simulink model "test_integration"  (R2022b)
settings: Solver=FixedStepAuto  StartTime=0.0  StopTime=240  FixedStep=0.1  RelTol=1e-3
(part 1 of 2)
settings Model: Creator=rosit  LastModifiedBy=cristian
settings ConfigComp: CovScope=ReferencedModels  CovIncludeTopModel=off  CovHTMLOptions=-sRT=1 -sVT=0 -aTS=1 -agT=1 -bRG=1 -bTC=1 -hTR=0 -nFC=0 -nFD=1 -scm=1 -bcm=1 -xEv=0 -xEM=0 -req=1  CovEnableCumulative=off

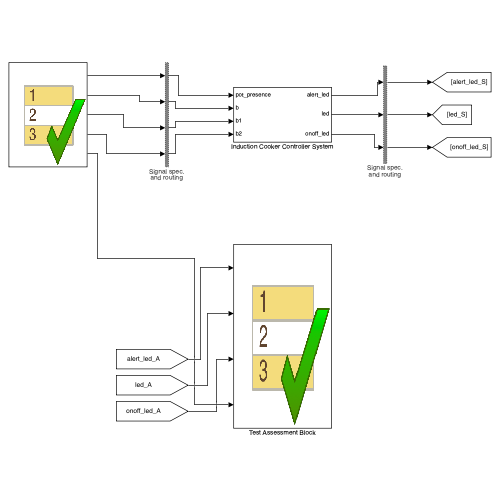
[thumbnail: Simulink's stored preview of the top-level diagram]
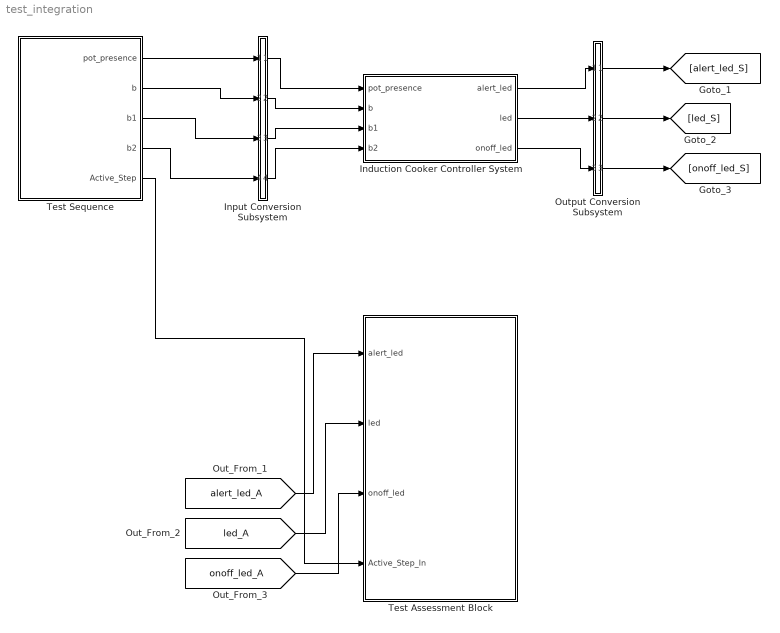
== system test_integration ==
  Induction Cooker Controller System : Subsystem
  Input Conversion Subsystem : Subsystem  Tag=__SLT_ICS__  Description=|
      | Signal spec.
      | and routing
      settings: AttributesFormatString=%<Description>
  Output Conversion Subsystem : Subsystem  Tag=__SLT_OCS__  Description=|
      | Signal spec.
      | and routing
      settings: AttributesFormatString=%<Description>
  Test Assessment Block : Test Sequence  Tag=__SLT_ASMT__  TreatAsAtomicUnit=on
  Test Sequence : Test Sequence  TreatAsAtomicUnit=on
  wires:
  [alert_led_A] -> Test Assessment Block/1(alert_led)
  [led_A] -> Test Assessment Block/2(led)
  [onoff_led_A] -> Test Assessment Block/3(onoff_led)
  Test Sequence/1(pot_presence) -> Input Conversion Subsystem/1(Inport_1)
  Test Sequence/2(b) -> Input Conversion Subsystem/2(Inport_2)
  Test Sequence/3(b1) -> Input Conversion Subsystem/3(Inport_3)
  Test Sequence/4(b2) -> Input Conversion Subsystem/4(Inport_4)
  Output Conversion Subsystem/1(Outport_1) -> [alert_led_S]
  Output Conversion Subsystem/2(Outport_2) -> [led_S]
  Output Conversion Subsystem/3(Outport_3) -> [onoff_led_S]
  Input Conversion Subsystem/1(Outport_1) -> Induction Cooker Controller System/1(pot_presence)
  Input Conversion Subsystem/2(Outport_2) -> Induction Cooker Controller System/2(b)
  Input Conversion Subsystem/3(Outport_3) -> Induction Cooker Controller System/3(b1)
  Input Conversion Subsystem/4(Outport_4) -> Induction Cooker Controller System/4(b2)
  Induction Cooker Controller System/1(alert_led) -> Output Conversion Subsystem/1(Inport_1)
  Induction Cooker Controller System/2(led) -> Output Conversion Subsystem/2(Inport_2)
  Induction Cooker Controller System/3(onoff_led) -> Output Conversion Subsystem/3(Inport_3)
  Test Sequence/5(Active_Step) -> Test Assessment Block/4(Active_Step_In)

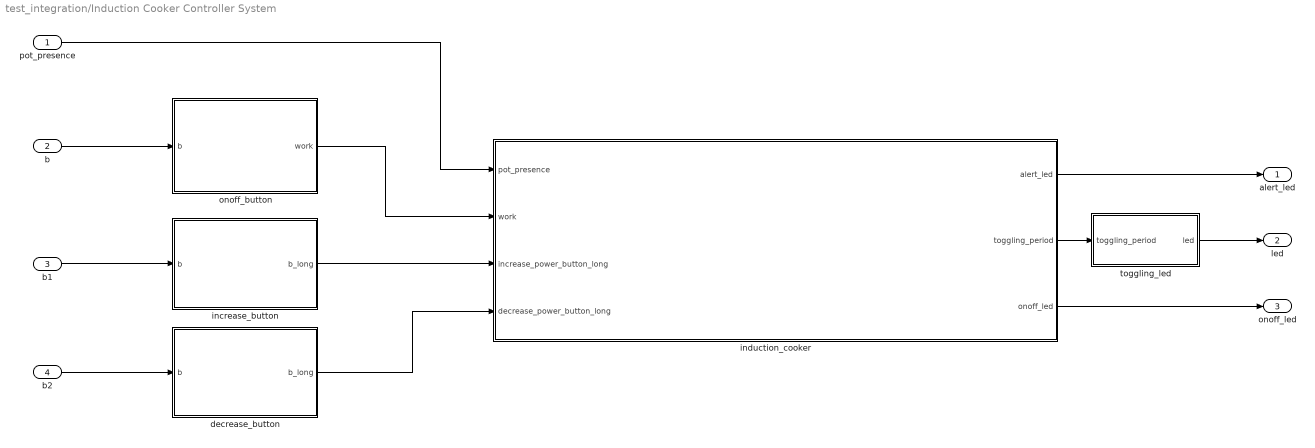
== system test_integration/Induction Cooker Controller System ==
  pot_presence : Inport
  b : Inport  Port=2
  b1 : Inport  Port=3
  b2 : Inport  Port=4
  decrease_button : Stateflow chart  TreatAsAtomicUnit=on
  increase_button : Stateflow chart  TreatAsAtomicUnit=on
  induction_cooker : Stateflow chart  TreatAsAtomicUnit=on
  onoff_button : Stateflow chart  TreatAsAtomicUnit=on
  toggling_led : Stateflow chart  TreatAsAtomicUnit=on
  alert_led : Outport
  led : Outport  Port=2
  onoff_led : Outport  Port=3
  wires:
  decrease_button/1(b_long) -> induction_cooker/4(decrease_power_button_long)
  increase_button/1(b_long) -> induction_cooker/3(increase_power_button_long)
  induction_cooker/2(toggling_period) -> toggling_led/1(toggling_period)
  toggling_led/1(led) -> led/1
  b1/1 -> increase_button/1(b)
  induction_cooker/3(onoff_led) -> onoff_led/1
  onoff_button/1(work) -> induction_cooker/2(work)
  b2/1 -> decrease_button/1(b)
  induction_cooker/1(alert_led) -> alert_led/1
  pot_presence/1 -> induction_cooker/1(pot_presence)
  b/1 -> onoff_button/1(b)

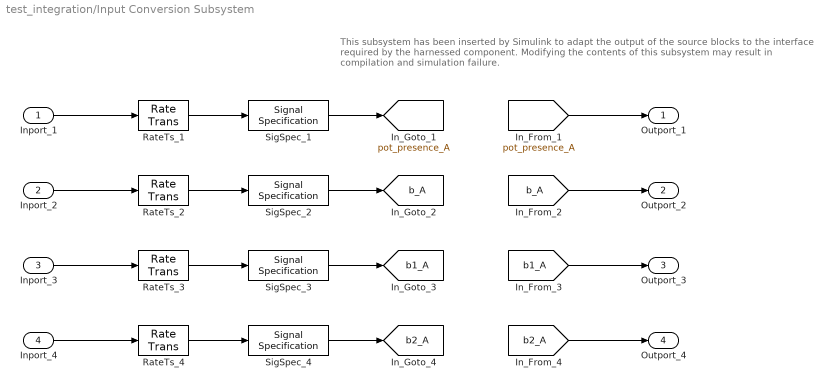
== system test_integration/Input Conversion Subsystem ==
  note: This subsystem has been inserted by Simulink to adapt the output of the source blocks to the interface required by the harnessed component.
      |  Modifying the contents of this subsystem may result in compilation and simulation failure.
  Inport_1 : Inport
  Inport_2 : Inport  Port=2
  Inport_3 : Inport  Port=3
  Inport_4 : Inport  Port=4
  RateTs_{1..4} (4 alike) : RateTransition  OutPortSampleTime=[-1, 0]
  SigSpec_{1..4} (4 alike) : SignalSpecification  OutDataTypeStr=boolean  Dimensions=[1]  SampleTime=[-1, 0]
  Outport_1 : Outport
  Outport_2 : Outport  Port=2
  Outport_3 : Outport  Port=3
  Outport_4 : Outport  Port=4
  tag scope: b1_A=global, b2_A=global, b_A=global, pot_presence_A=global
  wires:
  [pot_presence_A] -> Outport_1/1
  SigSpec_1/1 -> [pot_presence_A]
  RateTs_1/1 -> SigSpec_1/1
  Inport_1/1 -> RateTs_1/1
  [b_A] -> Outport_2/1
  SigSpec_2/1 -> [b_A]
  RateTs_2/1 -> SigSpec_2/1
  Inport_2/1 -> RateTs_2/1
  [b1_A] -> Outport_3/1
  SigSpec_3/1 -> [b1_A]
  RateTs_3/1 -> SigSpec_3/1
  Inport_3/1 -> RateTs_3/1
  [b2_A] -> Outport_4/1
  SigSpec_4/1 -> [b2_A]
  RateTs_4/1 -> SigSpec_4/1
  Inport_4/1 -> RateTs_4/1

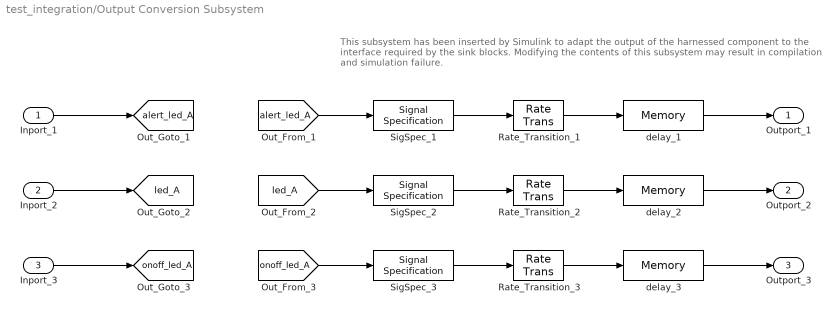
== system test_integration/Output Conversion Subsystem ==
  note: This subsystem has been inserted by Simulink to adapt the output of the harnessed component to the interface required by the sink blocks.
      |  Modifying the contents of this subsystem may result in compilation and simulation failure.
  Inport_1 : Inport
  Inport_2 : Inport  Port=2
  Inport_3 : Inport  Port=3
  Rate_Transition_1 : RateTransition  OutPortSampleTimeOpt=Inherit
  Rate_Transition_2 : RateTransition  OutPortSampleTimeOpt=Inherit
  Rate_Transition_3 : RateTransition  OutPortSampleTimeOpt=Inherit
  SigSpec_1 : SignalSpecification  OutDataTypeStr=boolean  Dimensions=[1]
  SigSpec_2 : SignalSpecification  OutDataTypeStr=boolean  Dimensions=[1]
  SigSpec_3 : SignalSpecification  OutDataTypeStr=boolean  Dimensions=[1]
  delay_1 : Memory
  delay_2 : Memory
  delay_3 : Memory
  Outport_1 : Outport
  Outport_2 : Outport  Port=2
  Outport_3 : Outport  Port=3
  tag scope: alert_led_A=global, led_A=global, onoff_led_A=global
  wires:
  Inport_1/1 -> [alert_led_A]
  [alert_led_A] -> SigSpec_1/1
  SigSpec_1/1 -> Rate_Transition_1/1
  Rate_Transition_1/1 -> delay_1/1
  delay_1/1 -> Outport_1/1
  Inport_2/1 -> [led_A]
  [led_A] -> SigSpec_2/1
  SigSpec_2/1 -> Rate_Transition_2/1
  Rate_Transition_2/1 -> delay_2/1
  delay_2/1 -> Outport_2/1
  Inport_3/1 -> [onoff_led_A]
  [onoff_led_A] -> SigSpec_3/1
  SigSpec_3/1 -> Rate_Transition_3/1
  Rate_Transition_3/1 -> delay_3/1
  delay_3/1 -> Outport_3/1

== stateflow chart test_integration/Induction Cooker Controller System/decrease_button ==
  note: Bottone a livelli, la pressione per un numero di secondi pari a DURATION permette di avere un uscita alta in maniera istantanea.
      | Per avere in output un valore PRESSED, è necessare lasciare il bottone e premere tra un output e l'altro.
  state Wait
    en: b_long = RELEASED
  state Pressed
    en: b_long = RELEASED;
    on after(DURATION,sec): b_long = PRESSED
  state LongPressed
    en: b_long = RELEASED
  (default) -> Wait
  Wait -> Pressed : [b == PRESSED]
  Pressed -> Wait [order 1] : [b == RELEASED]
  LongPressed -> Wait : [b == RELEASED]
  Pressed -> LongPressed [order 2] : [b_long == PRESSED && b == PRESSED]
  data: b_long output boolean size=1; PRESSED constant boolean size=1 =0; RELEASED constant boolean size=1 =1; b input boolean size=1; DURATION constant double size=1 =1

== stateflow chart test_integration/Induction Cooker Controller System/increase_button ==
  note: Bottone a livelli, la pressione per un numero di secondi pari a DURATION permette di avere un uscita alta in maniera istantanea.
      | Per avere in output un valore PRESSED, è necessare lasciare il bottone e premere tra un output e l'altro.
  state Wait
    en: b_long = RELEASED
  state Pressed
    en: b_long = RELEASED;
    on after(DURATION,sec): b_long = PRESSED
  state LongPressed
    en: b_long = RELEASED
  (default) -> Wait
  Wait -> Pressed : [b == PRESSED]
  Pressed -> Wait [order 1] : [b == RELEASED]
  LongPressed -> Wait : [b == RELEASED]
  Pressed -> LongPressed [order 2] : [b_long == PRESSED && b == PRESSED]
  data: b_long output boolean size=1; PRESSED constant boolean size=1 =0; RELEASED constant boolean size=1 =1; b input boolean size=1; DURATION constant double size=1 =1

== stateflow chart test_integration/Test Sequence ==
  settings: updateMethod=DISCRETE  sampleTime=0.1
  state IncreasePower
    state IP_Init
      %% Initialize data outputs.
      pot_presence = true;
      b = true;
      b1 = true;
      b2 = true;
      settings: description=Inizialmente il fornello è spento.
    state IP_TurnON
      pot_presence = true;
      b = false;
      b1 = true;
      b2 = true;
      settings: description=Accendiamo il fornello, premendo l'apposito pulsante di accensione. Il passaggio avveiene in maniera istantanea.
    state IP_IncreasePower300W
      pot_presence = false;
      b = true;
      b1 = false;
      b2 = true;
      settings: description=Posizioniamo la pentola ed accendiamo il fornello facendo pressione per 1 secondo sull'apposito pulsante di aumento potenza.
    state IP_Wait300W
      pot_presence = false;
      b = true;
      b1 = true;
      b2 = true;
      settings: description=Attendiamo 5 sec affinché il cambiamento diventi effettivo.
    state IP_Set300W
      pot_presence = false;
      b = true;
      b1 = true;
      b2 = true;
      settings: description=Il cambiamento di potenza viene effettuato.
    state IP_IncreasePower500W
      pot_presence = false;
      b = true;
      b1 = false;
      b2 = true;
      settings: description=Posizioniamo la pentola ed accendiamo il fornello facendo pressione per 1 secondo sull'apposito pulsante di aumento potenza.
    state IP_Wait500W
      pot_presence = false;
      b = true;
      b1 = true;
      b2 = true;
      settings: description=Attendiamo 5 sec affinché il cambiamento diventi effettivo.
    state IP_Set500W
      pot_presence = false;
      b = true;
      b1 = true;
      b2 = true;
      settings: description=Il cambiamento di potenza viene effettuato.
    state Void
    (default) -> IP_Init
    IP_Init -> IP_TurnON : [
        | true
        | ]
    IP_TurnON -> IP_IncreasePower300W : [
        | true
        | ]
    IP_IncreasePower300W -> IP_Wait300W : [
        | after(1+SamplePeriod,sec)
        | ]
    IP_Wait300W -> IP_Set300W : [
        | after(5-SamplePeriod,sec)
        | ]
    IP_Set300W -> IP_IncreasePower500W : [
        | true
        | ]
    IP_IncreasePower500W -> IP_Wait500W : [
        | after(1+SamplePeriod,sec)
        | ]
    IP_Wait500W -> IP_Set500W : [
        | after(5-SamplePeriod,sec)
        | ]
    IP_Set500W -> Void : [
        | true
        | ]
  state DecreasePower
    state DP_Init
      %% Initialize data outputs.
      pot_presence = true;
      b = true;
      b1 = true;
      b2 = true;
      settings: description=Inizialmente il fornello è spento.
    state DP_TurnON
      pot_presence = true;
      b = false;
      b1 = true;
      b2 = true;
      settings: description=Accendiamo il fornello, premendo l'apposito pulsante di accensione. Il passaggio avveiene in maniera istantanea.
    state DP_IncreasePower300W
      pot_presence = false;
      b = true;
      b1 = false;
      b2 = true;
      settings: description=Posizioniamo la pentola ed accendiamo il fornello facendo pressione per 1 secondo sull'apposito pulsante di aumento potenza.
    state DP_Wait300W
      pot_presence = false;
      b = true;
      b1 = true;
      b2 = true;
      settings: description=Attendiamo 5 sec affinché il cambiamento diventi effettivo.
    state DP_Set300W
      pot_presence = false;
      b = true;
      b1 = true;
      b2 = true;
      settings: description=Il cambiamento di potenza viene effettuato.
    state DP_DecreasePower0W
      pot_presence = false;
      b = true;
      b1 = true;
      b2 = false;
      settings: description=Facciamo pressione per 1 secondo sull'apposito pulsante di diminuzione di potenza.
    state DP_Wait0W
      pot_presence = false;
      b = true;
      b1 = true;
      b2 = true;
      settings: description=Attendiamo 5 sec affinché il cambiamento diventi effettivo.
    state DP_Set0W
      pot_presence = false;
      b = true;
      b1 = true;
      b2 = true;
      settings: description=Il cambiamento di potenza viene effettuato.
    state DP_void
    (default) -> DP_Init
    DP_Init -> DP_TurnON : [
        | true
        | ]
    DP_TurnON -> DP_IncreasePower300W : [
        | true
        | ]
    DP_IncreasePower300W -> DP_Wait300W : [
        | after(1+SamplePeriod,sec)
        | ]
    DP_Wait300W -> DP_Set300W : [
        | after(5-SamplePeriod,sec)
        | ]
    DP_Set300W -> DP_DecreasePower0W : [
        | true
        | ]
    DP_DecreasePower0W -> DP_Wait0W : [
        | after(1+SamplePeriod,sec)
        | ]
    DP_Wait0W -> DP_Set0W : [
        | after(5-SamplePeriod,sec)
        | ]
    DP_Set0W -> DP_void : [
        | true
        | ]
  state TurnOnOff
    state TO_Init
      %% Initialize data outputs.
      pot_presence = true;
      b = true;
      b1 = true;
      b2 = true;
      settings: description=All'inizio il fornello è spento e quindi anche il led di accensione.
    state TO_PowerOn
      pot_presence = true;
      b = false;
      b1 = true;
      b2 = true;
      settings: description=Dopodiché il bottone viene premuto ed il fornello si accende istantaneamente.
    state TO_Release
      pot_presence = true;
      b = true;
      b1 = true;
      b2 = true;
      settings: description=Quando il bottone viene rilasciato, il bottone ed il led di accensione sono entrambi accesi.
    state TO_PowerOff
      pot_presence = true;
      b = false;
      b1 = true;
      b2 = true;
      settings: description=Dopodiché il bottone viene ripremuto per la durata di un secondo ed il fornello, con il rispettivo led, vengono spenti.
    state TO_End
      pot_presence = true;
      b = true;
      b1 = true;
      b2 = true;
      settings: description=Infine il fornello è spento.
    state TO_Void
    (default) -> TO_Init
    TO_Init -> TO_PowerOn : [
        | true
        | ]
    TO_PowerOn -> TO_Release : [
        | true
        | ]
    TO_Release -> TO_PowerOff : [
        | true
        | ]
    TO_PowerOff -> TO_End : [
        | after(1+SamplePeriod,sec)
        | ]
    TO_End -> TO_Void : [
        | true
        | ]
  state PotRemovedWhileCooking
    state PR_Init
      %% Initialize data outputs.
      pot_presence = true;
      b = true;
      b1 = true;
      b2 = true;
      settings: description=inizialmente il fornello è spento.
    state PR_TurnOn
      pot_presence = true;
      b = false;
      b1 = true;
      b2 = true;
      settings: description=Accendiamo il fornello.
    state PR_IncreasePower300W
      pot_presence = false;
      b = true;
      b1 = false;
      b2 = true;
      settings: description=Pressione del bottone per incrementare la potenza da 0W a 300W.
    state PR_Wait300W
      pot_presence = false;
      b = true;
      b1 = true;
      b2 = true;
      settings: description=Attesa che il cambiamento di potenza sia effettivo per 5 sec.
    state PR_Set300W
      pot_presence = false;
      b = true;
      b1 = true;
      b2 = true;
      settings: description=Facciamo funzionare un po' il fornello.
    state PR_PotRemoved
      pot_presence = true;
      b = true;
      b1 = true;
      b2 = true;
      settings: description=|
          | La pentola viene rimossa dal fornello.
          | Si accende il led rosso.
    state PR_Alarm1
      pot_presence = true;
      b = true;
      b1 = true;
      b2 = true;
      settings: description=Il fornello è in stato di allarme, il led rosso è acceso
    state PR_PotPositioned
      pot_presence = false;
      b = true;
      b1 = true;
      b2 = true;
      settings: description=La pentola viene riposizionata, il led rosso si spegne, mentre il fornello continua a funzionare.
    state PR_ContinueWorking
      pot_presence = false;
      b = true;
      b1 = true;
      b2 = true;
      settings: description=Il fornello continua a funzionare normalmente per due secondi.
    state PR_PotRemoved2
      pot_presence = true;
      b = true;
      b1 = true;
      b2 = true;
      settings: description=La pentola viene rimossa e il fornello va immediatamente in tasto di allarme. Il led rosso si accende.
    state PR_Alarm2
      pot_presence = true;
      b = true;
      b1 = true;
      b2 = true;
      settings: description=Il fornello è instato di allarme, il led rosso è acceso.
    state PR_TimeElapsed
      pot_presence = true;
      b = true;
      b1 = true;
      b2 = true;
      settings: description=Il tempo di allarme è scaduto, il led rosso si è spento, il fornello è acceso, ma non sta funzionando (non è attivo).
    state PR_End
    (default) -> PR_Init
    PR_Init -> PR_TurnOn : [
        | true
        | ]
    PR_TurnOn -> PR_IncreasePower300W : [
        | true
        | ]
    PR_IncreasePower300W -> PR_Wait300W : [
        | after(1+SamplePeriod,sec)
        | ]
    PR_Wait300W -> PR_Set300W : [
        | after(5-SamplePeriod,sec)
        | ]
    PR_Set300W -> PR_PotRemoved : [
        | after(2*SamplePeriod,sec)
        | ]
    PR_PotRemoved -> PR_Alarm1 : [
        | true
        | ]
    PR_Alarm1 -> PR_PotPositioned : [
        | after(1-SamplePeriod,sec)
        | ]
    PR_PotPositioned -> PR_ContinueWorking : [
        | true
        | ]
    PR_ContinueWorking -> PR_PotRemoved2 : [
        | after(1-SamplePeriod,sec)
        | ]
    PR_PotRemoved2 -> PR_Alarm2 : [
        | true
        | ]
    PR_Alarm2 -> PR_TimeElapsed : [
        | after(10-SamplePeriod,sec)
        | ]
    PR_TimeElapsed -> PR_End : [
        | true
        | ]
  state IncreaseAndDecreaseBothPressed
    state BP_Init
      %% Initialize data outputs.
      pot_presence = true;
      b = true;
      b1 = true;
      b2 = true;
      settings: description=Inizialmente il fornello è spento, la pentola non è presente e tutti i led sono spenti.
    state BP_TurnOn
      pot_presence = true;
      b = false;
      b1 = true;
      b2 = true;
      settings: description=Il fornello viene acceso istantaneamente alla pressione dell'apposito bottone.
    state BP_IncreasePower300W
      pot_presence = false;
      b = true;
      b1 = false;
      b2 = true;
      settings: description=Viene richiesto l'incremento della potenza e quindi l'accensione del dispositivo.
    state BP_Wait300W
      pot_presence = false;
      b = true;
      b1 = true;
      b2 = true;
      settings: description=Il fornello si pone in attesa di una variazione della potenza erogata.
    state BP_Set300W
      pot_presence = false;
      b = true;
      b1 = true;
      b2 = true;
      settings: description=Cambio della potenza.
    state BP_BothButtonsPressed
      pot_presence = false;
      b = true;
      b1 = false;
      b2 = false;
      settings: description=Entrambi i bottoni di aumento e diminuzione della potenza vengono premuti.
    state BP_ButtonsReleased
      pot_presence = false;
      b = true;
      b1 = true;
      b2 = true;
      settings: description=I bottoni vengono rilasciati e ci aspettiamo che, poichè si è data priorità alle transizioni di diminuzione all'interno del chart, l'operazione che avrà la meglio è quella di decremento della potenza.
    state BP_SetNewPower
      pot_presence = false;
      b = true;
      b1 = true;
      b2 = true;
      settings: description=La nuova potenza viene confermata.
    state BP_Void
    (default) -> BP_Init
    BP_Init -> BP_TurnOn : [
        | true
        | ]
    BP_TurnOn -> BP_IncreasePower300W : [
        | true
        | ]
    BP_IncreasePower300W -> BP_Wait300W : [
        | after(1+SamplePeriod,sec)
        | ]
    BP_Wait300W -> BP_Set300W : [
        | after(5-SamplePeriod,sec)
        | ]
    BP_Set300W -> BP_BothButtonsPressed : [
        | true
        | ]
    BP_BothButtonsPressed -> BP_ButtonsReleased : [
        | after(1+SamplePeriod,sec)
        | ]
    BP_ButtonsReleased -> BP_SetNewPower : [
        | after(5-SamplePeriod,sec)
        | ]
    BP_SetNewPower -> BP_Void : [
        | true
        | ]
  state ChangePowerWhileWaiting
    state CP_Init
      %% Initialize data outputs.
      pot_presence = true;
      b = true;
      b1 = true;
      b2 = true;
      settings: description=Inizialmente il fornello è spento.
    state CP_TurnON
      pot_presence = true;
      b = false;
      b1 = true;
      b2 = true;
      settings: description=Accendiamo il fornello, premendo l'apposito pulsante di accensione. Il passaggio avveiene in maniera istantanea.
    state CP_IncreasePower300W
      pot_presence = false;
      b = true;
      b1 = false;
      b2 = true;
      settings: description=Posizioniamo la pentola ed accendiamo il fornello facendo pressione per 1 secondo sull'apposito pulsante di aumento potenza.
    state CP_Wait300W
      pot_presence = false;
      b = true;
      b1 = true;
      b2 = true;
      settings: description=Ci mettiamo in attesa di ulteriori cambiamenti di potenza per 5 secondi, ed effettivamente al secondo 3 avviene.
    state CP_IncreasePower500W
      pot_presence = false;
      b = true;
      b1 = false;
      b2 = true;
      settings: description=Facciamo pressione per 1 secondo dull'apposito pulsante di aumento potenza.
    state CP_Wait500W
      pot_presence = false;
      b = true;
      b1 = true;
      b2 = true;
      settings: description=Attendiamo 5 sec affinché il cambiamento diventi effettivo.
    state CP_Set500W
      pot_presence = false;
      b = true;
      b1 = true;
      b2 = true;
      settings: description=Il cambiamento di potenza viene effettuato.
    state CP_end
    (default) -> CP_Init
    CP_Init -> CP_TurnON : [
        | true
        | ]
    CP_TurnON -> CP_IncreasePower300W : [
        | true
        | ]
    CP_IncreasePower300W -> CP_Wait300W : [
        | after(1+SamplePeriod,sec)
        | ]
    CP_Wait300W -> CP_IncreasePower500W : [
        | after(3-SamplePeriod,sec)
        | ]
    CP_IncreasePower500W -> CP_Wait500W : [
        | after(1+SamplePeriod,sec)
        | ]
    CP_Wait500W -> CP_Set500W : [
        | after(5-SamplePeriod,sec)
        | ]
    CP_Set500W -> CP_end : [
        | true
        | ]
  (default) -> IncreasePower [order 1] : [Active_Scenario_Index == 1]
  (default) -> DecreasePower [order 2] : [Active_Scenario_Index == 2]
  (default) -> TurnOnOff [order 3] : [Active_Scenario_Index == 3]
  (default) -> PotRemovedWhileCooking [order 4] : [Active_Scenario_Index == 4]
  (default) -> IncreaseAndDecreaseBothPressed [order 5] : [Active_Scenario_Index == 5]
  (default) -> ChangePowerWhileWaiting [order 6] : {assert(Active_Scenario_Index == 6,'The value of Scenario Parameter ''Active_Scenario_Index'' is not valid. Use the index of the scenario to specify it.')}
  data: pot_presence output boolean size=[1]; b output boolean size=[1]; b1 output boolean size=[1]; b2 output boolean size=[1]; Active_Step output Enum: ActiveStepInt; SamplePeriod constant double =str2num(get_param('InductionCooker','FixedStep')); Active_Scenario_Index parameter =4

== stateflow chart test_integration/Induction Cooker Controller System/induction_cooker ==
  note: Il core del fornello è composto da un chart principale che oscilla tra uno stato ON ed uno stato OFF, a seconda dell'input work che ne indica in che stato di funzionamento deve essere (associato al bottone a livelli di on/off).
  state OFF
    en: onoff_led = LOW, alert_led = LOW,
    current_power = 0, toggling_period = TOGGLING_PERIOD_OFF
  note: Lo stato ON è composto da tre macchine parallele che gestiscono rispettivamente: cambiamento potenza, allarme e blink del led.
  state ON
    state LOGIC [parallel]
      settings: executionOrder=1
      note: In LOGIC, lo stato di ingresso è quello a 0W, in quanto appena accendiamo il fornello esso non è attivo.
          | Quando si riceve l'input di INCREASE o DECREASE button, si transita in uno stato che rappresenta una nuova potenza selezionata, dopo 5 secondi da un passaggio di stato la potenza reale diventerà quella associata allo stato correntemente attivo.
          | Quando una certa potenza viene selezionata, viene aggiornato il periodo di blink del power_led.
      state P0W
        state WAIT
        state SET
          en:
          current_power = 0, toggling_period = TOGGLING_PERIOD_0W
        note: Lo stato che rappresenta 0W gode della particolarità di poter fissare la potenza anche senza attendere i 5s, questo è possibile quando da uno stato gerarchicamente superiore o parallelo viene impostato current_power = 0W. Tale circostanza avviene sia all'avvio in cui non vi è necessità di attendere del tempo prima di impostare la potenza a 0W e sia nel momento in cui scatta l'allarme, in cui si disattiva il fornello istantaneamente.
        (default) -> ON.LOGIC.P0W.WAIT
        ON.LOGIC.P0W.WAIT -> ON.LOGIC.P0W.SET : [after(SET_POWER_PATIENCE,sec) || current_power == 0]
      note: Notiamo che in ogni stato di LOGIC, diverso da 0W, vi è una transizione associata al fatto che la variabile alarm assume valore HIGH, che ci riporta automaticamente nello stato 0W e fissa tale potenza come potenza corrente senza attendere i 10 secondi.
      state P1500W
        state WAIT
        state SET
          en:
          current_power = 1500, toggling_period = TOGGLING_PERIOD_1500W
        (default) -> ON.LOGIC.P1500W.WAIT
        ON.LOGIC.P1500W.WAIT -> ON.LOGIC.P1500W.SET : after(SET_POWER_PATIENCE,sec)
      state P300W
        state WAIT
        state SET
          en:
          current_power = 300, toggling_period = TOGGLING_PERIOD_300W
        (default) -> ON.LOGIC.P300W.WAIT
        ON.LOGIC.P300W.WAIT -> ON.LOGIC.P300W.SET : after(SET_POWER_PATIENCE,sec)
      state P1000W
        state WAIT
        state SET
          en:
          current_power = 1000, toggling_period = TOGGLING_PERIOD_1000W
        (default) -> ON.LOGIC.P1000W.WAIT
        ON.LOGIC.P1000W.WAIT -> ON.LOGIC.P1000W.SET : after(SET_POWER_PATIENCE,sec)
      state P500W
        state WAIT
        state SET
          en:
          current_power = 500, toggling_period = TOGGLING_PERIOD_500W
        (default) -> ON.LOGIC.P500W.WAIT
        ON.LOGIC.P500W.WAIT -> ON.LOGIC.P500W.SET : after(SET_POWER_PATIENCE,sec)
      (default) -> P0W
      P1500W -> P0W [order 2] : [alarm == HIGH]
      P0W -> P300W : [increase_power_button_long == PRESSED && pot_presence == PRESSED]
      P300W -> P0W [order 1] : [(alarm == HIGH) || (decrease_power_button_long == PRESSED && pot_presence == PRESSED)]
      P500W -> P0W [order 3] : [alarm == HIGH]
      P1000W -> P0W [order 3] : [alarm == HIGH]
      P500W -> P300W [order 1] : [decrease_power_button_long == PRESSED && pot_presence == PRESSED]
      P300W -> P500W [order 2] : [increase_power_button_long == PRESSED && pot_presence == PRESSED]
      P1500W -> P1000W [order 1] : [decrease_power_button_long == PRESSED && pot_presence == PRESSED]
      P1000W -> P1500W [order 2] : [increase_power_button_long == PRESSED && pot_presence == PRESSED]
      P500W -> P1000W [order 2] : [increase_power_button_long == PRESSED && pot_presence == PRESSED]
      P1000W -> P500W [order 1] : [decrease_power_button_long == PRESSED && pot_presence == PRESSED]
    state ALARM [parallel]
      settings: executionOrder=2
      state ACTIVE
        state QUIET
          en: alarm = LOW, alert_led = LOW
        state ALARM
          en: alert_led = HIGH
          on after(ALARM_PATIENCE,sec): alarm = HIGH; current_power = 0; toggling_period = TOGGLING_PERIOD_0W; alert_led = LOW;
        (default) -> QUIET
        QUIET -> ON.ALARM.ACTIVE.ALARM : [pot_presence == RELEASED]
        ON.ALARM.ACTIVE.ALARM -> QUIET : [pot_presence == PRESSED]
      state INACTIVE
        en:
        alarm = LOW,
        alert_led = LOW
      (default) -> INACTIVE
      INACTIVE -> ACTIVE : [current_power ~= 0]
      ACTIVE -> INACTIVE : [current_power == 0]
    state TOGGLING_LED [parallel] [commented out]
      note: In ogni stato di LOGIC, che rappresenta una specifica potenza, viene impostato un valore di periodo che indica ogni quanto il power_led (led giallo) lampeggia.
          | Infatti, tale macchina semplicemente rimbalza da uno stato all'altro accendendo e spegnendo il led.
      state LED_OFF [commented out]
        en: power_led=LOW;
      state LED_ON [commented out]
        en: power_led=HIGH;
      (default) -> LED_OFF [commented out]
      LED_OFF -> LED_ON [commented out] : [toggling_period>0 && after(toggling_period,sec)]
      LED_ON -> LED_OFF [commented out] : [after(toggling_period,sec)]
  note: Quando la macchina non è attiva (current_power = 0W), anche l'allarme è inattivo. All'attivazione del fornello corrisponde l'attivazione dell'allarme.
      | Nel momento in cui l'allarme è attivo e rileva una rimozione della pentola passa in uno stato ALARM che accende l'alert_led e dopo 10 secondi di permanenza disattiva il sistema portando LOGIC nello stato 0W, a meno di reinserimento pentola che riporta in uno stato QUIET.
  (default) -> OFF
  OFF -> ON : [work == HIGH]{onoff_led = HIGH}
  ON -> OFF : [work == LOW]
  data: pot_presence input boolean size=1; work input boolean size=1; alarm local boolean size=1; alert_led output boolean size=1; toggling_period output double size=1; onoff_led output boolean size=1; current_power local uint16 size=1; increase_power_button_long input boolean size=1; decrease_power_button_long input boolean size=1; HIGH constant boolean size=1 =1; PRESSED constant boolean size=1 =0; RELEASED constant boolean size=1 =1; LOW constant boolean size=1 =0; ALARM_PATIENCE constant double =10; TOGGLING_PERIOD_0W constant double =0; TOGGLING_PERIOD_300W constant double =2; TOGGLING_PERIOD_500W constant double =1; TOGGLING_PERIOD_1000W constant double =0.5; TOGGLING_PERIOD_1500W constant double =0.25; SET_POWER_PATIENCE local =5; TOGGLING_PERIOD_OFF constant double =0

== stateflow chart test_integration/Induction Cooker Controller System/onoff_button ==
  note: Stato di accensione del bottone onoff
  note: In questo stato il bottone può accendere la macchina
  state INACTIVE
    state Pressed
      en: work = HIGH
    state Wait
      en: work = LOW
    (default) -> INACTIVE.Wait
    INACTIVE.Wait -> INACTIVE.Pressed : [b == PRESSED]
  note: Stato di spegnimento del bottone onoff
  note: In questo stato il bottone può spengere la macchina
  state ACTIVE
    state Wait
      en:
      b_long = RELEASED
    state Pressed
      en:
      b_long = RELEASED;
      on after(DURATION,sec): b_long = PRESSED
    state LongPressed
      en: work = LOW;
    (default) -> ACTIVE.Wait
    ACTIVE.Wait -> ACTIVE.Pressed : [b == PRESSED]
    ACTIVE.Pressed -> ACTIVE.Wait [order 1] : [b == RELEASED]
    ACTIVE.Pressed -> LongPressed [order 2] : [b_long == PRESSED && b == PRESSED]
  note: Se il bottone viene premuto una sola volta, il sistema viene acceso.
      | Se il bottone viene premuto per 1 secondo, il sistema viene spento.
      | Una pressione prolungata senza rilascio del bottone, non causa un alternarsi di accensioni e spegnimenti continui.
  (default) -> INACTIVE
  INACTIVE.Pressed -> ACTIVE : [b == RELEASED]
  LongPressed -> INACTIVE : [b==RELEASED]
  data: PRESSED constant boolean size=1 =0; RELEASED constant boolean size=1 =1; b input boolean size=1; DURATION constant double size=1 =1; b_long local boolean size=1; HIGH constant boolean size=1 =1; LOW constant boolean size=1 =0; work output boolean size=1

== stateflow chart test_integration/Induction Cooker Controller System/toggling_led ==
  note: Lo spegnimento ha invece la priorità, appena ho periodo=0 spengo.
  state Off
    en: led = LOW
  state Blink_Off
    en:
    led = LOW
    period = toggling_period
  state Blink_On
    en:
    led = HIGH
    period = toggling_period
  note: L'utilizzo di una variabile di appoggio consente di gestire il caso in cui durante il blinking il periodo viene cambiato. Usando tale variabile, lo stato corrente viene termianto dopo un'attesa pari al vecchio periodo e dal nuovo stato vi sarà la variazione di periodo.
      | Ad esempio, se passo da 1s a 2s, ed attualmente il led è acceso, lo spegnerò terminando l'attesa di 1s e dal prossimo stato l'attesa sarà di 2s.
  (default) -> Off
  Blink_Off -> Off [order 1] : [toggling_period == 0]
  Blink_On -> Off [order 1] : [toggling_period == 0]
  Off -> Blink_On : [toggling_period ~= 0]
  Blink_On -> Blink_Off [order 2] : [after(period,sec)]
  Blink_Off -> Blink_On [order 2] : [after(period,sec)]
  data: toggling_period input double; led output boolean; HIGH constant boolean =1; LOW constant boolean =0; period local
